simulink model "case5"  (R2024b)
settings: Solver=FixedStepAuto  StartTime=0  StopTime=1  FixedStep=1e-7  RelTol=1e-3
values from neighbouring files (symbols this model uses):
  SG_D_1_D = 0.01056    [IEEE9_case_parameters.m]    (also in case1_parameters.m; case2_parameters.m; case3_parameters.m; case4_parameters.m)
  SG_D_1_EnableSaturation = 0    [IEEE9_case_parameters.m]    (also in case1_parameters.m; case2_parameters.m; case3_parameters.m; case4_parameters.m)
  SG_D_1_f0 = 60    [IEEE9_case_parameters.m]    (also in case1_parameters.m; case2_parameters.m; case3_parameters.m; case4_parameters.m)
  SG_D_1_H = 7.5    [IEEE9_case_parameters.m]    (also in case1_parameters.m; case2_parameters.m; case3_parameters.m; case4_parameters.m)
  SG_D_1_K_A = 20    [IEEE9_case_parameters.m]    (also in case1_parameters.m; case2_parameters.m; case3_parameters.m; case4_parameters.m)
  SG_D_1_K_E = 1.000000e+1    (= 10)    [IEEE9_case_parameters.m]    (also in case1_parameters.m; case2_parameters.m; case3_parameters.m; case4_parameters.m)
  SG_D_1_K_F = 2.363    [IEEE9_case_parameters.m]    (also in case1_parameters.m; case2_parameters.m; case3_parameters.m; case4_parameters.m)
  SG_D_1_K_s = 0.5    [IEEE9_case_parameters.m]    (also in case1_parameters.m = 5; case2_parameters.m = 5; case3_parameters.m = 5; case4_parameters.m = 5)
  SG_D_1_R_a = 0.001088    [IEEE9_case_parameters.m]    (also in case1_parameters.m; case2_parameters.m; case3_parameters.m; case4_parameters.m)
  SG_D_1_S_A = 1    [IEEE9_case_parameters.m]    (also in case1_parameters.m; case2_parameters.m; case3_parameters.m; case4_parameters.m)
  SG_D_1_S_B = 0.103    [IEEE9_case_parameters.m]    (also in case1_parameters.m; case2_parameters.m; case3_parameters.m; case4_parameters.m)
  SG_D_1_S_N = 10.659857    [IEEE9_case_parameters.m]    (also in case1_parameters.m; case2_parameters.m; case3_parameters.m; case4_parameters.m)
  SG_D_1_SpeedPara = 200    [IEEE9_case_parameters.m]    (also in case1_parameters.m; case2_parameters.m; case3_parameters.m; case4_parameters.m)
  SG_D_1_T_0 = 0.720173    [IEEE9_case_parameters.m]    (also in case1_parameters.m = 0.755522; case2_parameters.m = 0.808931; case3_parameters.m = 0.869402; case4_parameters.m = 0.729316)
  SG_D_1_T_1 = 0.3    [IEEE9_case_parameters.m]    (also in case1_parameters.m; case2_parameters.m; case3_parameters.m; case4_parameters.m)
  SG_D_1_T_2 = 0.05    [IEEE9_case_parameters.m]    (also in case1_parameters.m; case2_parameters.m; case3_parameters.m; case4_parameters.m)
  SG_D_1_T_3 = 0.02    [IEEE9_case_parameters.m]    (also in case1_parameters.m; case2_parameters.m; case3_parameters.m; case4_parameters.m)
  SG_D_1_T_4 = 0.005    [IEEE9_case_parameters.m]    (also in case1_parameters.m; case2_parameters.m; case3_parameters.m; case4_parameters.m)
  SG_D_1_T_A = 0.02    [IEEE9_case_parameters.m]    (also in case1_parameters.m; case2_parameters.m; case3_parameters.m; case4_parameters.m)
  SG_D_1_T_dd = 8.000000e+0    (= 8)    [IEEE9_case_parameters.m]    (also in case1_parameters.m; case2_parameters.m; case3_parameters.m; case4_parameters.m)
  SG_D_1_T_ddd = 0.04    [IEEE9_case_parameters.m]    (also in case1_parameters.m; case2_parameters.m; case3_parameters.m; case4_parameters.m)
  SG_D_1_T_E = 0.314    [IEEE9_case_parameters.m]    (also in case1_parameters.m; case2_parameters.m; case3_parameters.m; case4_parameters.m)
  SG_D_1_T_F = 0.35    [IEEE9_case_parameters.m]    (also in case1_parameters.m; case2_parameters.m; case3_parameters.m; case4_parameters.m)
  SG_D_1_T_qd = 0.8    [IEEE9_case_parameters.m]    (also in case1_parameters.m; case2_parameters.m; case3_parameters.m; case4_parameters.m)
  SG_D_1_T_qdd = 0.02    [IEEE9_case_parameters.m]    (also in case1_parameters.m; case2_parameters.m; case3_parameters.m; case4_parameters.m)
  SG_D_1_T_speed = 0.1    [IEEE9_case_parameters.m]    (also in case1_parameters.m = 200; case2_parameters.m = 200; case3_parameters.m = 200; case4_parameters.m = 200)
  SG_D_1_T_w = 0.5    [IEEE9_case_parameters.m]    (also in case1_parameters.m; case2_parameters.m; case3_parameters.m; case4_parameters.m)
  SG_D_1_V_ref = 1.990276    [IEEE9_case_parameters.m]    (also in case1_parameters.m = 2.042296; case2_parameters.m = 2.051388; case3_parameters.m = 2.089584; case4_parameters.m = 2.01845)
  SG_D_1_w_ref = 376.991118    [IEEE9_case_parameters.m]    (also in case1_parameters.m; case2_parameters.m; case3_parameters.m; case4_parameters.m)
  SG_D_1_wb = 6.000000e+1    (= 60)    [IEEE9_case_parameters.m]    (also in case1_parameters.m; case2_parameters.m; case3_parameters.m; case4_parameters.m)
  SG_D_1_x_d = 1.9    [IEEE9_case_parameters.m]    (also in case1_parameters.m; case2_parameters.m; case3_parameters.m; case4_parameters.m)
  SG_D_1_x_dd = 0.302    [IEEE9_case_parameters.m]    (also in case1_parameters.m; case2_parameters.m; case3_parameters.m; case4_parameters.m)
  SG_D_1_x_ddd = 0.204    [IEEE9_case_parameters.m]    (also in case1_parameters.m; case2_parameters.m; case3_parameters.m; case4_parameters.m)
  SG_D_1_x_l = 0.05    [IEEE9_case_parameters.m]    (also in case1_parameters.m; case2_parameters.m; case3_parameters.m; case4_parameters.m)
  SG_D_1_x_q = 1.3    [IEEE9_case_parameters.m]    (also in case1_parameters.m; case2_parameters.m; case3_parameters.m; case4_parameters.m)
  SG_D_1_x_qd = 0.5    [IEEE9_case_parameters.m]    (also in case1_parameters.m; case2_parameters.m; case3_parameters.m; case4_parameters.m)
  SG_D_1_x_qdd = 0.3    [IEEE9_case_parameters.m]    (also in case1_parameters.m; case2_parameters.m; case3_parameters.m; case4_parameters.m)
  SG_D_2_D = 0.02    [IEEE9_case_parameters.m]    (also in case1_parameters.m; case2_parameters.m; case3_parameters.m; case4_parameters.m)
  SG_D_2_EnableSaturation = 0    [IEEE9_case_parameters.m]    (also in case1_parameters.m; case2_parameters.m; case3_parameters.m; case4_parameters.m)
  SG_D_2_f0 = 60    [IEEE9_case_parameters.m]    (also in case1_parameters.m; case2_parameters.m; case3_parameters.m; case4_parameters.m)
  SG_D_2_H = 8.000000e+0    (= 8)    [IEEE9_case_parameters.m]    (also in case1_parameters.m; case2_parameters.m; case3_parameters.m; case4_parameters.m)
  SG_D_2_K_A = 20    [IEEE9_case_parameters.m]    (also in case1_parameters.m; case2_parameters.m; case3_parameters.m; case4_parameters.m)
  SG_D_2_K_E = 1.000000e+1    (= 10)    [IEEE9_case_parameters.m]    (also in case1_parameters.m; case2_parameters.m; case3_parameters.m; case4_parameters.m)
  SG_D_2_K_F = 2.363    [IEEE9_case_parameters.m]    (also in case1_parameters.m; case2_parameters.m; case3_parameters.m; case4_parameters.m)
  SG_D_2_K_s = 0.5    [IEEE9_case_parameters.m]    (also in case1_parameters.m = 4; case2_parameters.m = 4; case3_parameters.m = 4; case4_parameters.m = 4)
  SG_D_2_R_a = 0.001088    [IEEE9_case_parameters.m]    (also in case1_parameters.m; case2_parameters.m; case3_parameters.m; case4_parameters.m)
  SG_D_2_S_A = 1    [IEEE9_case_parameters.m]    (also in case1_parameters.m; case2_parameters.m; case3_parameters.m; case4_parameters.m)
  SG_D_2_S_B = 0.103    [IEEE9_case_parameters.m]    (also in case1_parameters.m; case2_parameters.m; case3_parameters.m; case4_parameters.m)
  SG_D_2_S_N = 10.659857    [IEEE9_case_parameters.m]    (also in case1_parameters.m; case2_parameters.m; case3_parameters.m; case4_parameters.m)
  SG_D_2_SpeedPara = 200    [IEEE9_case_parameters.m]    (also in case1_parameters.m; case2_parameters.m; case3_parameters.m; case4_parameters.m)
  SG_D_2_T_0 = 1.632913    [IEEE9_case_parameters.m]    (also in case1_parameters.m = 1.632925; case2_parameters.m = 1.632915; case3_parameters.m = 1.632914; case4_parameters.m = 1.632927)
  SG_D_2_T_1 = 0.2    [IEEE9_case_parameters.m]    (also in case1_parameters.m; case2_parameters.m; case3_parameters.m; case4_parameters.m)
  SG_D_2_T_2 = 0.05    [IEEE9_case_parameters.m]    (also in case1_parameters.m; case2_parameters.m; case3_parameters.m; case4_parameters.m)
  SG_D_2_T_3 = 0.02    [IEEE9_case_parameters.m]    (also in case1_parameters.m; case2_parameters.m; case3_parameters.m; case4_parameters.m)
  SG_D_2_T_4 = 0.005    [IEEE9_case_parameters.m]    (also in case1_parameters.m; case2_parameters.m; case3_parameters.m; case4_parameters.m)
  SG_D_2_T_A = 0.02    [IEEE9_case_parameters.m]    (also in case1_parameters.m; case2_parameters.m; case3_parameters.m; case4_parameters.m)
  SG_D_2_T_dd = 7.9    [IEEE9_case_parameters.m]    (also in case1_parameters.m; case2_parameters.m; case3_parameters.m; case4_parameters.m)
  SG_D_2_T_ddd = 0.04    [IEEE9_case_parameters.m]    (also in case1_parameters.m; case2_parameters.m; case3_parameters.m; case4_parameters.m)
  SG_D_2_T_E = 0.314    [IEEE9_case_parameters.m]    (also in case1_parameters.m; case2_parameters.m; case3_parameters.m; case4_parameters.m)
  SG_D_2_T_F = 0.35    [IEEE9_case_parameters.m]    (also in case1_parameters.m; case2_parameters.m; case3_parameters.m; case4_parameters.m)
  SG_D_2_T_qd = 0.8    [IEEE9_case_parameters.m]    (also in case1_parameters.m; case2_parameters.m; case3_parameters.m; case4_parameters.m)
  SG_D_2_T_qdd = 0.015    [IEEE9_case_parameters.m]    (also in case1_parameters.m; case2_parameters.m; case3_parameters.m; case4_parameters.m)
  SG_D_2_T_speed = 0.1    [IEEE9_case_parameters.m]    (also in case1_parameters.m = 150; case2_parameters.m = 150; case3_parameters.m = 150; case4_parameters.m = 150)
  SG_D_2_T_w = 0.35    [IEEE9_case_parameters.m]    (also in case1_parameters.m; case2_parameters.m; case3_parameters.m; case4_parameters.m)
  SG_D_2_V_ref = 2.58547    [IEEE9_case_parameters.m]    (also in case1_parameters.m = 2.597896; case2_parameters.m = 2.587136; case3_parameters.m = 2.586042; case4_parameters.m = 2.599679)
  SG_D_2_w_ref = 376.991118    [IEEE9_case_parameters.m]    (also in case1_parameters.m; case2_parameters.m; case3_parameters.m; case4_parameters.m)
  SG_D_2_wb = 6.000000e+1    (= 60)    [IEEE9_case_parameters.m]    (also in case1_parameters.m; case2_parameters.m; case3_parameters.m; case4_parameters.m)
  SG_D_2_x_d = 1.8    [IEEE9_case_parameters.m]    (also in case1_parameters.m; case2_parameters.m; case3_parameters.m; case4_parameters.m)
  SG_D_2_x_dd = 0.302    [IEEE9_case_parameters.m]    (also in case1_parameters.m; case2_parameters.m; case3_parameters.m; case4_parameters.m)
  SG_D_2_x_ddd = 0.204    [IEEE9_case_parameters.m]    (also in case1_parameters.m; case2_parameters.m; case3_parameters.m; case4_parameters.m)
  SG_D_2_x_l = 0.05    [IEEE9_case_parameters.m]    (also in case1_parameters.m; case2_parameters.m; case3_parameters.m; case4_parameters.m)
  SG_D_2_x_q = 1.25    [IEEE9_case_parameters.m]    (also in case1_parameters.m; case2_parameters.m; case3_parameters.m; case4_parameters.m)
  SG_D_2_x_qd = 0.5    [IEEE9_case_parameters.m]    (also in case1_parameters.m; case2_parameters.m; case3_parameters.m; case4_parameters.m)
  SG_D_2_x_qdd = 0.3    [IEEE9_case_parameters.m]    (also in case1_parameters.m; case2_parameters.m; case3_parameters.m; case4_parameters.m)
  SG_D_3_D = 0.02    [IEEE9_case_parameters.m]    (also in case1_parameters.m; case2_parameters.m; case3_parameters.m; case4_parameters.m)
  SG_D_3_EnableSaturation = 0    [IEEE9_case_parameters.m]    (also in case1_parameters.m; case2_parameters.m; case3_parameters.m; case4_parameters.m)
  SG_D_3_f0 = 60    [IEEE9_case_parameters.m]    (also in case1_parameters.m; case2_parameters.m; case3_parameters.m; case4_parameters.m)
  SG_D_3_H = 7.7    [IEEE9_case_parameters.m]    (also in case1_parameters.m; case2_parameters.m; case3_parameters.m; case4_parameters.m)
  SG_D_3_K_A = 20    [IEEE9_case_parameters.m]    (also in case1_parameters.m; case2_parameters.m; case3_parameters.m; case4_parameters.m)
  SG_D_3_K_E = 1.000000e+1    (= 10)    [IEEE9_case_parameters.m]    (also in case1_parameters.m; case2_parameters.m; case3_parameters.m; case4_parameters.m)
  SG_D_3_K_F = 2.363    [IEEE9_case_parameters.m]    (also in case1_parameters.m; case2_parameters.m; case3_parameters.m; case4_parameters.m)
  SG_D_3_K_s = 0.2    [IEEE9_case_parameters.m]    (also in case1_parameters.m = 2; case2_parameters.m = 2; case3_parameters.m = 2; case4_parameters.m = 2)
  SG_D_3_R_a = 0.001088    [IEEE9_case_parameters.m]    (also in case1_parameters.m; case2_parameters.m; case3_parameters.m; case4_parameters.m)
  SG_D_3_S_A = 1    [IEEE9_case_parameters.m]    (also in case1_parameters.m; case2_parameters.m; case3_parameters.m; case4_parameters.m)
  SG_D_3_S_B = 0.103    [IEEE9_case_parameters.m]    (also in case1_parameters.m; case2_parameters.m; case3_parameters.m; case4_parameters.m)
  SG_D_3_S_N = 10.659857    [IEEE9_case_parameters.m]    (also in case1_parameters.m; case2_parameters.m; case3_parameters.m; case4_parameters.m)
  SG_D_3_SpeedPara = 200    [IEEE9_case_parameters.m]    (also in case1_parameters.m; case2_parameters.m; case3_parameters.m; case4_parameters.m)
  SG_D_3_T_0 = 0.850788    [IEEE9_case_parameters.m]    (also in case1_parameters.m = 0.850786; case2_parameters.m = 0.850787; case3_parameters.m; case4_parameters.m = 0.850786)
  SG_D_3_T_1 = 0.2    [IEEE9_case_parameters.m]    (also in case1_parameters.m; case2_parameters.m; case3_parameters.m; case4_parameters.m)
  SG_D_3_T_2 = 0.05    [IEEE9_case_parameters.m]    (also in case1_parameters.m; case2_parameters.m; case3_parameters.m; case4_parameters.m)
  SG_D_3_T_3 = 0.02    [IEEE9_case_parameters.m]    (also in case1_parameters.m; case2_parameters.m; case3_parameters.m; case4_parameters.m)
  SG_D_3_T_4 = 0.005    [IEEE9_case_parameters.m]    (also in case1_parameters.m; case2_parameters.m; case3_parameters.m; case4_parameters.m)
  SG_D_3_T_A = 0.02    [IEEE9_case_parameters.m]    (also in case1_parameters.m; case2_parameters.m; case3_parameters.m; case4_parameters.m)
  SG_D_3_T_dd = 8.1    [IEEE9_case_parameters.m]    (also in case1_parameters.m; case2_parameters.m; case3_parameters.m; case4_parameters.m)
  SG_D_3_T_ddd = 0.04    [IEEE9_case_parameters.m]    (also in case1_parameters.m; case2_parameters.m; case3_parameters.m; case4_parameters.m)
  SG_D_3_T_E = 0.314    [IEEE9_case_parameters.m]    (also in case1_parameters.m; case2_parameters.m; case3_parameters.m; case4_parameters.m)
  SG_D_3_T_F = 0.35    [IEEE9_case_parameters.m]    (also in case1_parameters.m; case2_parameters.m; case3_parameters.m; case4_parameters.m)
  SG_D_3_T_qd = 0.8    [IEEE9_case_parameters.m]    (also in case1_parameters.m; case2_parameters.m; case3_parameters.m; case4_parameters.m)
  SG_D_3_T_qdd = 0.015    [IEEE9_case_parameters.m]    (also in case1_parameters.m; case2_parameters.m; case3_parameters.m; case4_parameters.m)
  SG_D_3_T_speed = 0.1    [IEEE9_case_parameters.m]    (also in case1_parameters.m = 180; case2_parameters.m = 180; case3_parameters.m = 180; case4_parameters.m = 180)
  SG_D_3_T_w = 0.4    [IEEE9_case_parameters.m]    (also in case1_parameters.m; case2_parameters.m; case3_parameters.m; case4_parameters.m)
  SG_D_3_V_ref = 1.892727    [IEEE9_case_parameters.m]    (also in case1_parameters.m = 1.906439; case2_parameters.m = 1.895535; case3_parameters.m = 1.892105; case4_parameters.m = 1.906598)
  SG_D_3_w_ref = 376.991118    [IEEE9_case_parameters.m]    (also in case1_parameters.m; case2_parameters.m; case3_parameters.m; case4_parameters.m)
  SG_D_3_wb = 6.000000e+1    (= 60)    [IEEE9_case_parameters.m]    (also in case1_parameters.m; case2_parameters.m; case3_parameters.m; case4_parameters.m)
  SG_D_3_x_d = 1.85    [IEEE9_case_parameters.m]    (also in case1_parameters.m; case2_parameters.m; case3_parameters.m; case4_parameters.m)
  SG_D_3_x_dd = 0.302    [IEEE9_case_parameters.m]    (also in case1_parameters.m; case2_parameters.m; case3_parameters.m; case4_parameters.m)
  SG_D_3_x_ddd = 0.204    [IEEE9_case_parameters.m]    (also in case1_parameters.m; case2_parameters.m; case3_parameters.m; case4_parameters.m)
  SG_D_3_x_l = 0.05    [IEEE9_case_parameters.m]    (also in case1_parameters.m; case2_parameters.m; case3_parameters.m; case4_parameters.m)
  SG_D_3_x_q = 1.2    [IEEE9_case_parameters.m]    (also in case1_parameters.m; case2_parameters.m; case3_parameters.m; case4_parameters.m)
  SG_D_3_x_qd = 0.5    [IEEE9_case_parameters.m]    (also in case1_parameters.m; case2_parameters.m; case3_parameters.m; case4_parameters.m)
  SG_D_3_x_qdd = 0.3    [IEEE9_case_parameters.m]    (also in case1_parameters.m; case2_parameters.m; case3_parameters.m; case4_parameters.m)
(part 2 of 12)

== system case5/SG_D_2 ==
  v_d_SG_D_2 : Inport
  v_q_SG_D_2 : Inport  Port=2
  E_fd_SG_D_2 : Integrator  InitialCondition=3.1862497744439606
  Px_1_SG_D_2 : Integrator  InitialCondition=0.0
  Px_2_SG_D_2 : Integrator  InitialCondition=0.0
  Px_3_SG_D_2 : Integrator  InitialCondition=6.670039757612852e-24
  R_f_SG_D_2 : Integrator  InitialCondition=21.5117377628888
  T_e_SG_D_2_block : Subsystem
  T_m_SG_D_2 : Integrator  InitialCondition=1.6329204678673217
  V_f_SG_D_2 : Integrator  InitialCondition=31.862497744439608
  d_E_fd_SG_D_2_block : Subsystem
  d_Px_1_SG_D_2_block : Subsystem
  d_Px_2_SG_D_2_block : Subsystem
  d_Px_3_SG_D_2_block : Subsystem
  d_R_f_SG_D_2_block : Subsystem
  d_T_m_SG_D_2_block : Subsystem
  d_V_f_SG_D_2_block : Subsystem
  d_psi_1d_SG_D_2_block : Subsystem
  d_psi_d_SG_D_2_block : Subsystem
  d_psi_fd_SG_D_2_block : Subsystem
  d_psi_gq_SG_D_2_block : Subsystem
  d_psi_kq_SG_D_2_block : Subsystem
  d_psi_q_SG_D_2_block : Subsystem
  d_theta_SG_D_2_block : Subsystem
  d_w_SG_D_2_block : Subsystem
  i_d_SG_D_2_block : Subsystem
  i_q_SG_D_2_block : Subsystem
  psi_1d_SG_D_2 : Integrator  InitialCondition=0.5852448096125112
  psi_d_SG_D_2 : Integrator  InitialCondition=0.5109303820458982
  psi_fd_SG_D_2 : Integrator  InitialCondition=0.95978952454824
  psi_gq_SG_D_2 : Integrator  InitialCondition=0.5170107087646497
  psi_kq_SG_D_2 : Integrator  InitialCondition=-0.8272171340234395
  psi_q_SG_D_2 : Integrator  InitialCondition=-0.8616845146077495
  theta_SG_D_2 : Integrator  InitialCondition=1.2193477459639033
  theta_SG_D_2_out_block : Subsystem
  w_SG_D_2 : Integrator  InitialCondition=376.99111843077515
  w_SG_D_2_out_block : Subsystem
  i_d_SG_D_2 : Outport
  i_q_SG_D_2 : Outport  Port=2
  T_e_SG_D_2 : Outport  Port=3
  w_SG_D_2_out : Outport  Port=4
  theta_SG_D_2_out : Outport  Port=5
  wires:
  d_T_m_SG_D_2_block/1(Blockout_d_T_m_SG_D_2_8be19) -> T_m_SG_D_2/1
  T_e_SG_D_2_block/1(Blockout_T_e_SG_D_2_32ea4) -> T_e_SG_D_2/1
  d_Px_2_SG_D_2_block/1(Blockout_d_Px_2_SG_D_2_04e36) -> Px_2_SG_D_2/1
  w_SG_D_2/1 -> d_psi_q_SG_D_2_block/9(State_w_SG_D_2_ff297), d_psi_d_SG_D_2_block/9(State_w_SG_D_2_93911), d_w_SG_D_2_block/1(State_w_SG_D_2_6739b), d_V_f_SG_D_2_block/8(State_w_SG_D_2_0ea60), d_V_f_SG_D_2_block/13(State_w_SG_D_2_f8832), d_theta_SG_D_2_block/1(State_w_SG_D_2_4ff61), d_T_m_SG_D_2_block/1(State_w_SG_D_2_ee856), d_Px_2_SG_D_2_block/4(State_w_SG_D_2_c4bce), d_Px_3_SG_D_2_block/6(State_w_SG_D_2_e9070), d_Px_1_SG_D_2_block/2(State_w_SG_D_2_0a872), w_SG_D_2_out_block/1(State_w_SG_D_2_5e653)
  d_Px_1_SG_D_2_block/1(Blockout_d_Px_1_SG_D_2_3a836) -> Px_1_SG_D_2/1
  d_theta_SG_D_2_block/1(Blockout_d_theta_SG_D_2_f9fe2) -> theta_SG_D_2/1
  psi_q_SG_D_2/1 -> d_psi_d_SG_D_2_block/8(State_psi_q_SG_D_2_39081), d_psi_gq_SG_D_2_block/9(State_psi_q_SG_D_2_8da15), d_psi_kq_SG_D_2_block/5(State_psi_q_SG_D_2_342e1), d_psi_gq_SG_D_2_block/6(State_psi_q_SG_D_2_ffa91), d_w_SG_D_2_block/6(State_psi_q_SG_D_2_d0bfc), d_V_f_SG_D_2_block/7(State_psi_q_SG_D_2_3f571), d_V_f_SG_D_2_block/11(State_psi_q_SG_D_2_64f5f), i_q_SG_D_2_block/3(State_psi_q_SG_D_2_28683), d_w_SG_D_2_block/7(State_psi_q_SG_D_2_59cd6), d_psi_q_SG_D_2_block/3(State_psi_q_SG_D_2_48ee2), T_e_SG_D_2_block/4(State_psi_q_SG_D_2_7d7d0), T_e_SG_D_2_block/5(State_psi_q_SG_D_2_860cc), i_d_SG_D_2_block/3(State_psi_q_SG_D_2_2fd58)
  w_SG_D_2_out_block/1(Blockout_w_SG_D_2_out_edd03) -> w_SG_D_2_out/1
  d_Px_3_SG_D_2_block/1(Blockout_d_Px_3_SG_D_2_0e921) -> Px_3_SG_D_2/1
  psi_gq_SG_D_2/1 -> d_psi_q_SG_D_2_block/1(State_psi_gq_SG_D_2_56d9a), d_psi_gq_SG_D_2_block/1(State_psi_gq_SG_D_2_87c46), d_psi_gq_SG_D_2_block/2(State_psi_gq_SG_D_2_c98fa), d_psi_gq_SG_D_2_block/4(State_psi_gq_SG_D_2_58af0), d_psi_kq_SG_D_2_block/3(State_psi_gq_SG_D_2_50e2d), d_w_SG_D_2_block/4(State_psi_gq_SG_D_2_c0fca), d_psi_gq_SG_D_2_block/7(State_psi_gq_SG_D_2_c3a0a), i_d_SG_D_2_block/1(State_psi_gq_SG_D_2_2f279), d_psi_kq_SG_D_2_block/1(State_psi_gq_SG_D_2_a995b), i_q_SG_D_2_block/1(State_psi_gq_SG_D_2_27a63), d_V_f_SG_D_2_block/9(State_psi_gq_SG_D_2_79d5b), T_e_SG_D_2_block/2(State_psi_gq_SG_D_2_1f7cf)
  psi_fd_SG_D_2/1 -> d_psi_fd_SG_D_2_block/2(State_psi_fd_SG_D_2_52249), d_psi_fd_SG_D_2_block/4(State_psi_fd_SG_D_2_bd521), d_psi_fd_SG_D_2_block/10(State_psi_fd_SG_D_2_29cbb), d_psi_fd_SG_D_2_block/7(State_psi_fd_SG_D_2_2448d), d_psi_d_SG_D_2_block/3(State_psi_fd_SG_D_2_ff9ed), d_V_f_SG_D_2_block/6(State_psi_fd_SG_D_2_d94f6), d_psi_1d_SG_D_2_block/2(State_psi_fd_SG_D_2_ecfb2), i_d_SG_D_2_block/7(State_psi_fd_SG_D_2_ae8c9), d_w_SG_D_2_block/10(State_psi_fd_SG_D_2_d0345), d_psi_1d_SG_D_2_block/5(State_psi_fd_SG_D_2_f55be), i_q_SG_D_2_block/7(State_psi_fd_SG_D_2_80ec4), T_e_SG_D_2_block/8(State_psi_fd_SG_D_2_f288a)
  psi_kq_SG_D_2/1 -> d_V_f_SG_D_2_block/10(State_psi_kq_SG_D_2_dc614), d_w_SG_D_2_block/5(State_psi_kq_SG_D_2_46ea8), d_psi_gq_SG_D_2_block/5(State_psi_kq_SG_D_2_220dd), d_psi_kq_SG_D_2_block/4(State_psi_kq_SG_D_2_80926), i_d_SG_D_2_block/2(State_psi_kq_SG_D_2_3a555), d_psi_gq_SG_D_2_block/8(State_psi_kq_SG_D_2_f5814), d_psi_q_SG_D_2_block/2(State_psi_kq_SG_D_2_66775), i_q_SG_D_2_block/2(State_psi_kq_SG_D_2_d20f4), d_psi_gq_SG_D_2_block/3(State_psi_kq_SG_D_2_803f1), T_e_SG_D_2_block/3(State_psi_kq_SG_D_2_b1f64), d_psi_kq_SG_D_2_block/2(State_psi_kq_SG_D_2_e8f3b)
  psi_1d_SG_D_2/1 -> d_psi_fd_SG_D_2_block/3(State_psi_1d_SG_D_2_569a8), d_psi_fd_SG_D_2_block/5(State_psi_1d_SG_D_2_de869), d_psi_fd_SG_D_2_block/8(State_psi_1d_SG_D_2_50b72), d_psi_d_SG_D_2_block/1(State_psi_1d_SG_D_2_04eff), d_psi_1d_SG_D_2_block/3(State_psi_1d_SG_D_2_31dd9), d_w_SG_D_2_block/8(State_psi_1d_SG_D_2_f1571), d_V_f_SG_D_2_block/4(State_psi_1d_SG_D_2_e8660), i_d_SG_D_2_block/5(State_psi_1d_SG_D_2_aa18d), i_q_SG_D_2_block/5(State_psi_1d_SG_D_2_19eb0), T_e_SG_D_2_block/6(State_psi_1d_SG_D_2_4989b), d_psi_1d_SG_D_2_block/1(State_psi_1d_SG_D_2_febab)
  Px_1_SG_D_2/1 -> d_Px_3_SG_D_2_block/4(State_Px_1_SG_D_2_820be), d_Px_1_SG_D_2_block/1(State_Px_1_SG_D_2_dcfec), d_Px_3_SG_D_2_block/5(State_Px_1_SG_D_2_81adf), d_Px_2_SG_D_2_block/3(State_Px_1_SG_D_2_6b838), d_Px_2_SG_D_2_block/2(State_Px_1_SG_D_2_e7928)
  theta_SG_D_2/1 -> d_psi_d_SG_D_2_block/5(State_theta_SG_D_2_47dce), d_psi_d_SG_D_2_block/7(State_theta_SG_D_2_18c28), i_d_SG_D_2_block/4(State_theta_SG_D_2_e2546), i_q_SG_D_2_block/4(State_theta_SG_D_2_24bbd), d_psi_q_SG_D_2_block/5(State_theta_SG_D_2_953f6), i_q_SG_D_2_block/8(State_theta_SG_D_2_e7cf1), i_d_SG_D_2_block/8(State_theta_SG_D_2_a5f3d), d_psi_q_SG_D_2_block/7(State_theta_SG_D_2_428e6), theta_SG_D_2_out_block/1(State_theta_SG_D_2_369d6)
  Px_2_SG_D_2/1 -> d_Px_3_SG_D_2_block/2(State_Px_2_SG_D_2_ea741), d_Px_2_SG_D_2_block/1(State_Px_2_SG_D_2_3d84e), d_Px_3_SG_D_2_block/3(State_Px_2_SG_D_2_55edc)
  v_d_SG_D_2/1 -> d_psi_d_SG_D_2_block/4(Input_v_d_SG_D_2_e8182), d_psi_q_SG_D_2_block/4(Input_v_d_SG_D_2_6ca72)
  i_d_SG_D_2_block/1(Blockout_i_d_SG_D_2_72f47) -> i_d_SG_D_2/1
  psi_d_SG_D_2/1 -> d_psi_fd_SG_D_2_block/6(State_psi_d_SG_D_2_2ae43), d_psi_d_SG_D_2_block/2(State_psi_d_SG_D_2_38234), d_psi_1d_SG_D_2_block/4(State_psi_d_SG_D_2_bbb49), d_V_f_SG_D_2_block/12(State_psi_d_SG_D_2_2ef51), d_V_f_SG_D_2_block/5(State_psi_d_SG_D_2_250ba), d_psi_q_SG_D_2_block/8(State_psi_d_SG_D_2_a68ec), d_w_SG_D_2_block/9(State_psi_d_SG_D_2_c4658), i_d_SG_D_2_block/6(State_psi_d_SG_D_2_3866e), T_e_SG_D_2_block/1(State_psi_d_SG_D_2_8764f), d_w_SG_D_2_block/3(State_psi_d_SG_D_2_c40be), d_psi_fd_SG_D_2_block/9(State_psi_d_SG_D_2_60bb1), i_q_SG_D_2_block/6(State_psi_d_SG_D_2_881d1), T_e_SG_D_2_block/7(State_psi_d_SG_D_2_cc96c)
  d_V_f_SG_D_2_block/1(Blockout_d_V_f_SG_D_2_8ab92) -> V_f_SG_D_2/1
  v_q_SG_D_2/1 -> d_psi_d_SG_D_2_block/6(Input_v_q_SG_D_2_617bb), d_psi_q_SG_D_2_block/6(Input_v_q_SG_D_2_c1f9e)
  T_m_SG_D_2/1 -> d_T_m_SG_D_2_block/2(State_T_m_SG_D_2_0b68a), d_w_SG_D_2_block/2(State_T_m_SG_D_2_a5b2e)
  R_f_SG_D_2/1 -> d_R_f_SG_D_2_block/2(State_R_f_SG_D_2_625bf), d_V_f_SG_D_2_block/2(State_R_f_SG_D_2_30619)
  theta_SG_D_2_out_block/1(Blockout_theta_SG_D_2_out_abd77) -> theta_SG_D_2_out/1
  d_psi_kq_SG_D_2_block/1(Blockout_d_psi_kq_SG_D_2_70fc6) -> psi_kq_SG_D_2/1
  d_R_f_SG_D_2_block/1(Blockout_d_R_f_SG_D_2_818dd) -> R_f_SG_D_2/1
  d_psi_gq_SG_D_2_block/1(Blockout_d_psi_gq_SG_D_2_29e5c) -> psi_gq_SG_D_2/1
  d_psi_1d_SG_D_2_block/1(Blockout_d_psi_1d_SG_D_2_44b96) -> psi_1d_SG_D_2/1
  d_psi_q_SG_D_2_block/1(Blockout_d_psi_q_SG_D_2_3921f) -> psi_q_SG_D_2/1
  d_psi_d_SG_D_2_block/1(Blockout_d_psi_d_SG_D_2_c5ec0) -> psi_d_SG_D_2/1
  d_w_SG_D_2_block/1(Blockout_d_w_SG_D_2_3d116) -> w_SG_D_2/1
  i_q_SG_D_2_block/1(Blockout_i_q_SG_D_2_ddca7) -> i_q_SG_D_2/1
  V_f_SG_D_2/1 -> d_V_f_SG_D_2_block/14(State_V_f_SG_D_2_95214), d_E_fd_SG_D_2_block/2(State_V_f_SG_D_2_4e077)
  Px_3_SG_D_2/1 -> d_V_f_SG_D_2_block/3(State_Px_3_SG_D_2_b4828), d_Px_3_SG_D_2_block/1(State_Px_3_SG_D_2_615b8)
  d_E_fd_SG_D_2_block/1(Blockout_d_E_fd_SG_D_2_55c73) -> E_fd_SG_D_2/1
  E_fd_SG_D_2/1 -> d_V_f_SG_D_2_block/1(State_E_fd_SG_D_2_ced48), d_R_f_SG_D_2_block/1(State_E_fd_SG_D_2_65d60), d_E_fd_SG_D_2_block/1(State_E_fd_SG_D_2_808fd), d_psi_fd_SG_D_2_block/1(State_E_fd_SG_D_2_4bfea)
  d_psi_fd_SG_D_2_block/1(Blockout_d_psi_fd_SG_D_2_6ca49) -> psi_fd_SG_D_2/1

== system case5/SG_D_3 ==
  v_d_SG_D_3 : Inport
  v_q_SG_D_3 : Inport  Port=2
  E_fd_SG_D_3 : Integrator  InitialCondition=1.7984887709053456
  Px_1_SG_D_3 : Integrator  InitialCondition=0.0
  Px_2_SG_D_3 : Integrator  InitialCondition=0.0
  Px_3_SG_D_3 : Integrator  InitialCondition=-1.4673797984671398e-24
  R_f_SG_D_3 : Integrator  InitialCondition=12.142368473283806
  T_e_SG_D_3_block : Subsystem
  T_m_SG_D_3 : Integrator  InitialCondition=0.8507866955563819
  V_f_SG_D_3 : Integrator  InitialCondition=17.984887709053456
  d_E_fd_SG_D_3_block : Subsystem
  d_Px_1_SG_D_3_block : Subsystem
  d_Px_2_SG_D_3_block : Subsystem
  d_Px_3_SG_D_3_block : Subsystem
  d_R_f_SG_D_3_block : Subsystem
  d_T_m_SG_D_3_block : Subsystem
  d_V_f_SG_D_3_block : Subsystem
  d_psi_1d_SG_D_3_block : Subsystem
  d_psi_d_SG_D_3_block : Subsystem
  d_psi_fd_SG_D_3_block : Subsystem
  d_psi_gq_SG_D_3_block : Subsystem
  d_psi_kq_SG_D_3_block : Subsystem
  d_psi_q_SG_D_3_block : Subsystem
  d_theta_SG_D_3_block : Subsystem
  d_w_SG_D_3_block : Subsystem
  i_d_SG_D_3_block : Subsystem
  i_q_SG_D_3_block : Subsystem
  psi_1d_SG_D_3 : Integrator  InitialCondition=0.7206007980275798
  psi_d_SG_D_3 : Integrator  InitialCondition=0.6906594654476417
  psi_fd_SG_D_3 : Integrator  InitialCondition=0.8715051142304671
  psi_gq_SG_D_3 : Integrator  InitialCondition=0.4226007274570196
  psi_kq_SG_D_3 : Integrator  InitialCondition=-0.6942726236793892
  psi_q_SG_D_3 : Integrator  InitialCondition=-0.7244583899263193
  theta_SG_D_3 : Integrator  InitialCondition=0.9043269566391599
  theta_SG_D_3_out_block : Subsystem
  w_SG_D_3 : Integrator  InitialCondition=376.99111843077515
  w_SG_D_3_out_block : Subsystem
  i_d_SG_D_3 : Outport
  i_q_SG_D_3 : Outport  Port=2
  T_e_SG_D_3 : Outport  Port=3
  w_SG_D_3_out : Outport  Port=4
  theta_SG_D_3_out : Outport  Port=5
  wires:
  d_Px_1_SG_D_3_block/1(Blockout_d_Px_1_SG_D_3_9be4e) -> Px_1_SG_D_3/1
  w_SG_D_3/1 -> d_psi_d_SG_D_3_block/9(State_w_SG_D_3_5916e), d_w_SG_D_3_block/1(State_w_SG_D_3_c3b06), d_V_f_SG_D_3_block/8(State_w_SG_D_3_90604), d_psi_q_SG_D_3_block/9(State_w_SG_D_3_7587a), d_V_f_SG_D_3_block/13(State_w_SG_D_3_d21e8), d_theta_SG_D_3_block/1(State_w_SG_D_3_3c4ab), d_T_m_SG_D_3_block/1(State_w_SG_D_3_0ca8a), d_Px_1_SG_D_3_block/2(State_w_SG_D_3_220ce), d_Px_2_SG_D_3_block/4(State_w_SG_D_3_ac5cc), d_Px_3_SG_D_3_block/6(State_w_SG_D_3_03b1d), w_SG_D_3_out_block/1(State_w_SG_D_3_fee15)
  d_T_m_SG_D_3_block/1(Blockout_d_T_m_SG_D_3_d3830) -> T_m_SG_D_3/1
  d_w_SG_D_3_block/1(Blockout_d_w_SG_D_3_cf3fb) -> w_SG_D_3/1
  Px_1_SG_D_3/1 -> d_Px_3_SG_D_3_block/4(State_Px_1_SG_D_3_769ed), d_Px_2_SG_D_3_block/3(State_Px_1_SG_D_3_6c166), d_Px_2_SG_D_3_block/2(State_Px_1_SG_D_3_ebea2), d_Px_3_SG_D_3_block/5(State_Px_1_SG_D_3_ab3a0), d_Px_1_SG_D_3_block/1(State_Px_1_SG_D_3_e9303)
  d_theta_SG_D_3_block/1(Blockout_d_theta_SG_D_3_6d326) -> theta_SG_D_3/1
  Px_2_SG_D_3/1 -> d_Px_2_SG_D_3_block/1(State_Px_2_SG_D_3_b50b4), d_Px_3_SG_D_3_block/2(State_Px_2_SG_D_3_8f252), d_Px_3_SG_D_3_block/3(State_Px_2_SG_D_3_5d3da)
  d_Px_3_SG_D_3_block/1(Blockout_d_Px_3_SG_D_3_07f5b) -> Px_3_SG_D_3/1
  R_f_SG_D_3/1 -> d_V_f_SG_D_3_block/2(State_R_f_SG_D_3_65c10), d_R_f_SG_D_3_block/2(State_R_f_SG_D_3_2ac4f)
  w_SG_D_3_out_block/1(Blockout_w_SG_D_3_out_017ab) -> w_SG_D_3_out/1
  d_Px_2_SG_D_3_block/1(Blockout_d_Px_2_SG_D_3_d6435) -> Px_2_SG_D_3/1
  T_m_SG_D_3/1 -> d_T_m_SG_D_3_block/2(State_T_m_SG_D_3_db6e5), d_w_SG_D_3_block/2(State_T_m_SG_D_3_e3476)
  v_d_SG_D_3/1 -> d_psi_q_SG_D_3_block/4(Input_v_d_SG_D_3_84d49), d_psi_d_SG_D_3_block/4(Input_v_d_SG_D_3_606f6)
  v_q_SG_D_3/1 -> d_psi_d_SG_D_3_block/6(Input_v_q_SG_D_3_a4294), d_psi_q_SG_D_3_block/6(Input_v_q_SG_D_3_69553)
  psi_kq_SG_D_3/1 -> d_psi_q_SG_D_3_block/2(State_psi_kq_SG_D_3_924ec), d_psi_gq_SG_D_3_block/3(State_psi_kq_SG_D_3_58aa9), d_psi_gq_SG_D_3_block/5(State_psi_kq_SG_D_3_80c97), d_psi_kq_SG_D_3_block/4(State_psi_kq_SG_D_3_7e333), d_w_SG_D_3_block/5(State_psi_kq_SG_D_3_92701), d_V_f_SG_D_3_block/10(State_psi_kq_SG_D_3_31833), i_d_SG_D_3_block/2(State_psi_kq_SG_D_3_2d375), d_psi_kq_SG_D_3_block/2(State_psi_kq_SG_D_3_1fc99), T_e_SG_D_3_block/3(State_psi_kq_SG_D_3_f2804), i_q_SG_D_3_block/2(State_psi_kq_SG_D_3_73f11), d_psi_gq_SG_D_3_block/8(State_psi_kq_SG_D_3_d3364)
  theta_SG_D_3/1 -> d_psi_d_SG_D_3_block/5(State_theta_SG_D_3_c5e42), d_psi_q_SG_D_3_block/7(State_theta_SG_D_3_ee4f0), i_d_SG_D_3_block/8(State_theta_SG_D_3_5a6b6), i_q_SG_D_3_block/4(State_theta_SG_D_3_ec54c), i_d_SG_D_3_block/4(State_theta_SG_D_3_03d7d), d_psi_q_SG_D_3_block/5(State_theta_SG_D_3_74150), i_q_SG_D_3_block/8(State_theta_SG_D_3_27a42), d_psi_d_SG_D_3_block/7(State_theta_SG_D_3_aedc7), theta_SG_D_3_out_block/1(State_theta_SG_D_3_f776d)
  psi_d_SG_D_3/1 -> d_psi_fd_SG_D_3_block/6(State_psi_d_SG_D_3_99e22), d_psi_fd_SG_D_3_block/9(State_psi_d_SG_D_3_9a2c9), d_psi_d_SG_D_3_block/2(State_psi_d_SG_D_3_d393d), d_psi_q_SG_D_3_block/8(State_psi_d_SG_D_3_b8185), d_psi_1d_SG_D_3_block/4(State_psi_d_SG_D_3_3e3a9), d_w_SG_D_3_block/9(State_psi_d_SG_D_3_9af62), d_V_f_SG_D_3_block/12(State_psi_d_SG_D_3_26750), i_d_SG_D_3_block/6(State_psi_d_SG_D_3_22276), d_V_f_SG_D_3_block/5(State_psi_d_SG_D_3_3db68), i_q_SG_D_3_block/6(State_psi_d_SG_D_3_fdaf0), d_w_SG_D_3_block/3(State_psi_d_SG_D_3_b825f), T_e_SG_D_3_block/1(State_psi_d_SG_D_3_0515e), T_e_SG_D_3_block/7(State_psi_d_SG_D_3_355d2)
  d_psi_kq_SG_D_3_block/1(Blockout_d_psi_kq_SG_D_3_acb7b) -> psi_kq_SG_D_3/1
  psi_1d_SG_D_3/1 -> d_psi_fd_SG_D_3_block/3(State_psi_1d_SG_D_3_a842a), d_psi_fd_SG_D_3_block/5(State_psi_1d_SG_D_3_8aaf0), d_psi_fd_SG_D_3_block/8(State_psi_1d_SG_D_3_7f19e), d_psi_d_SG_D_3_block/1(State_psi_1d_SG_D_3_2013b), d_w_SG_D_3_block/8(State_psi_1d_SG_D_3_df021), d_V_f_SG_D_3_block/4(State_psi_1d_SG_D_3_fdc7a), i_d_SG_D_3_block/5(State_psi_1d_SG_D_3_ba81f), i_q_SG_D_3_block/5(State_psi_1d_SG_D_3_88e27), d_psi_1d_SG_D_3_block/1(State_psi_1d_SG_D_3_3b403), T_e_SG_D_3_block/6(State_psi_1d_SG_D_3_44396), d_psi_1d_SG_D_3_block/3(State_psi_1d_SG_D_3_4c72e)
  psi_q_SG_D_3/1 -> d_psi_d_SG_D_3_block/8(State_psi_q_SG_D_3_01c82), d_psi_gq_SG_D_3_block/6(State_psi_q_SG_D_3_d87f8), d_psi_gq_SG_D_3_block/9(State_psi_q_SG_D_3_0f8a4), d_psi_kq_SG_D_3_block/5(State_psi_q_SG_D_3_1522f), d_psi_q_SG_D_3_block/3(State_psi_q_SG_D_3_33284), d_V_f_SG_D_3_block/7(State_psi_q_SG_D_3_72b18), d_w_SG_D_3_block/6(State_psi_q_SG_D_3_c3d2e), d_V_f_SG_D_3_block/11(State_psi_q_SG_D_3_0b65f), i_d_SG_D_3_block/3(State_psi_q_SG_D_3_70eb0), i_q_SG_D_3_block/3(State_psi_q_SG_D_3_60de2), T_e_SG_D_3_block/4(State_psi_q_SG_D_3_52c06), d_w_SG_D_3_block/7(State_psi_q_SG_D_3_f932d), T_e_SG_D_3_block/5(State_psi_q_SG_D_3_d7233)
  psi_fd_SG_D_3/1 -> d_psi_fd_SG_D_3_block/2(State_psi_fd_SG_D_3_7ac4b), d_psi_fd_SG_D_3_block/4(State_psi_fd_SG_D_3_12a65), d_psi_fd_SG_D_3_block/10(State_psi_fd_SG_D_3_0d84b), d_psi_1d_SG_D_3_block/5(State_psi_fd_SG_D_3_649d9), d_psi_fd_SG_D_3_block/7(State_psi_fd_SG_D_3_2014a), d_w_SG_D_3_block/10(State_psi_fd_SG_D_3_b5ce7), d_V_f_SG_D_3_block/6(State_psi_fd_SG_D_3_cd25d), i_q_SG_D_3_block/7(State_psi_fd_SG_D_3_58217), d_psi_1d_SG_D_3_block/2(State_psi_fd_SG_D_3_f9b6a), d_psi_d_SG_D_3_block/3(State_psi_fd_SG_D_3_0e180), T_e_SG_D_3_block/8(State_psi_fd_SG_D_3_44178), i_d_SG_D_3_block/7(State_psi_fd_SG_D_3_ca9c0)
  psi_gq_SG_D_3/1 -> d_psi_q_SG_D_3_block/1(State_psi_gq_SG_D_3_1dddd), d_psi_gq_SG_D_3_block/1(State_psi_gq_SG_D_3_42abb), d_psi_gq_SG_D_3_block/2(State_psi_gq_SG_D_3_81b5d), d_psi_gq_SG_D_3_block/4(State_psi_gq_SG_D_3_55563), d_psi_kq_SG_D_3_block/3(State_psi_gq_SG_D_3_b2b08), d_w_SG_D_3_block/4(State_psi_gq_SG_D_3_617ad), d_V_f_SG_D_3_block/9(State_psi_gq_SG_D_3_47fb2), d_psi_gq_SG_D_3_block/7(State_psi_gq_SG_D_3_b3e08), i_d_SG_D_3_block/1(State_psi_gq_SG_D_3_83e92), i_q_SG_D_3_block/1(State_psi_gq_SG_D_3_e58b5), T_e_SG_D_3_block/2(State_psi_gq_SG_D_3_1cc94), d_psi_kq_SG_D_3_block/1(State_psi_gq_SG_D_3_4cb6a)
  theta_SG_D_3_out_block/1(Blockout_theta_SG_D_3_out_a9243) -> theta_SG_D_3_out/1
  d_V_f_SG_D_3_block/1(Blockout_d_V_f_SG_D_3_d48b4) -> V_f_SG_D_3/1
  i_d_SG_D_3_block/1(Blockout_i_d_SG_D_3_8b105) -> i_d_SG_D_3/1
  d_psi_d_SG_D_3_block/1(Blockout_d_psi_d_SG_D_3_27069) -> psi_d_SG_D_3/1
  i_q_SG_D_3_block/1(Blockout_i_q_SG_D_3_d37fb) -> i_q_SG_D_3/1
  d_psi_q_SG_D_3_block/1(Blockout_d_psi_q_SG_D_3_a4a1c) -> psi_q_SG_D_3/1
  d_R_f_SG_D_3_block/1(Blockout_d_R_f_SG_D_3_894a9) -> R_f_SG_D_3/1
  d_psi_1d_SG_D_3_block/1(Blockout_d_psi_1d_SG_D_3_0c79f) -> psi_1d_SG_D_3/1
  T_e_SG_D_3_block/1(Blockout_T_e_SG_D_3_5900b) -> T_e_SG_D_3/1
  d_psi_gq_SG_D_3_block/1(Blockout_d_psi_gq_SG_D_3_5066e) -> psi_gq_SG_D_3/1
  V_f_SG_D_3/1 -> d_V_f_SG_D_3_block/14(State_V_f_SG_D_3_66c81), d_E_fd_SG_D_3_block/2(State_V_f_SG_D_3_2af07)
  Px_3_SG_D_3/1 -> d_V_f_SG_D_3_block/3(State_Px_3_SG_D_3_a594e), d_Px_3_SG_D_3_block/1(State_Px_3_SG_D_3_2f57b)
  d_E_fd_SG_D_3_block/1(Blockout_d_E_fd_SG_D_3_8336f) -> E_fd_SG_D_3/1
  E_fd_SG_D_3/1 -> d_V_f_SG_D_3_block/1(State_E_fd_SG_D_3_5ffef), d_E_fd_SG_D_3_block/1(State_E_fd_SG_D_3_d3096), d_psi_fd_SG_D_3_block/1(State_E_fd_SG_D_3_c498c), d_R_f_SG_D_3_block/1(State_E_fd_SG_D_3_8b5d7)
  d_psi_fd_SG_D_3_block/1(Blockout_d_psi_fd_SG_D_3_9596e) -> psi_fd_SG_D_3/1

== system case5/AC_1/d_id_line_1_4_block ==
  note: d_id_line_1_4 in case5
      | $376.991118430775\,\mathrm{iq}_{\mathrm{line},1,4}+6332.81249201072\,\mathrm{vd}_{\mathrm{bus},1}-6332.81249201072\,\mathrm{vd}_{\mathrm{bus},4}$
      | Automatically generated on 2025-10-31 19:14:13 .
  State_iq_line_1_4_f9009 : Inport
  State_vd_bus_1_aee9d : Inport  Port=2
  State_vd_bus_4_1db4d : Inport  Port=3
  Add_ead1a : Sum
  Constant_376.991118430775_7df71 : Constant  Value=376.991118430775
  Constant_6332.81249201072_2a037 : Constant  Value=6332.81249201072
  Constant_6332.81249201072_2c4bb : Constant  Value=6332.81249201072
  Product_04931 : Product
  Product_4f94b : Product
  Product_907b6 : Product
  Subtract_c8ec4 : Sum  Inputs=+-
  Blockout_d_id_line_1_4_69e37 : Outport
  wires:
  Constant_376.991118430775_7df71/1 -> Product_907b6/1
  Product_4f94b/1 -> Add_ead1a/2
  State_iq_line_1_4_f9009/1 -> Product_907b6/2
  Subtract_c8ec4/1 -> Blockout_d_id_line_1_4_69e37/1
  Constant_6332.81249201072_2c4bb/1 -> Product_4f94b/1
  Product_907b6/1 -> Add_ead1a/1
  State_vd_bus_1_aee9d/1 -> Product_4f94b/2
  Constant_6332.81249201072_2a037/1 -> Product_04931/1
  State_vd_bus_4_1db4d/1 -> Product_04931/2
  Add_ead1a/1 -> Subtract_c8ec4/1
  Product_04931/1 -> Subtract_c8ec4/2

== system case5/AC_1/d_id_line_3_6_block ==
  note: d_id_line_3_6 in case5
      | $376.991118430775\,\mathrm{iq}_{\mathrm{line},3,6}+6224.74401945081\,\mathrm{vd}_{\mathrm{bus},3}-6224.74401945081\,\mathrm{vd}_{\mathrm{bus},6}$
      | Automatically generated on 2025-10-31 19:14:22 .
  State_iq_line_3_6_0028c : Inport
  State_vd_bus_3_b4f76 : Inport  Port=2
  State_vd_bus_6_aaa66 : Inport  Port=3
  Add_fe0f0 : Sum
  Constant_376.991118430775_66f8f : Constant  Value=376.991118430775
  Constant_6224.74401945081_f6c00 : Constant  Value=6224.74401945081
  Constant_6224.74401945081_fa8d3 : Constant  Value=6224.74401945081
  Product_20f8b : Product
  Product_2217c : Product
  Product_6d514 : Product
  Subtract_a8b68 : Sum  Inputs=+-
  Blockout_d_id_line_3_6_09483 : Outport
  wires:
  State_vd_bus_3_b4f76/1 -> Product_2217c/2
  Constant_376.991118430775_66f8f/1 -> Product_6d514/1
  Product_2217c/1 -> Add_fe0f0/2
  State_iq_line_3_6_0028c/1 -> Product_6d514/2
  Constant_6224.74401945081_f6c00/1 -> Product_2217c/1
  Product_6d514/1 -> Add_fe0f0/1
  Constant_6224.74401945081_fa8d3/1 -> Product_20f8b/1
  State_vd_bus_6_aaa66/1 -> Product_20f8b/2
  Add_fe0f0/1 -> Subtract_a8b68/1
  Product_20f8b/1 -> Subtract_a8b68/2
  Subtract_a8b68/1 -> Blockout_d_id_line_3_6_09483/1

== system case5/AC_1/d_id_line_4_5_block ==
  note: d_id_line_4_5 in case5
      | $376.991118430775\,\mathrm{iq}_{\mathrm{line},4,5}-65.6746171008477\,\mathrm{id}_{\mathrm{line},4,5}+3964.89129934584\,\mathrm{vd}_{\mathrm{bus},4}-3964.89129934584\,\mathrm{vd}_{\mathrm{bus},5}$
      | Automatically generated on 2025-10-31 19:14:16 .
  State_id_line_4_5_17bd4 : Inport
  State_iq_line_4_5_655b9 : Inport  Port=2
  State_vd_bus_4_6c299 : Inport  Port=3
  State_vd_bus_5_8ddf9 : Inport  Port=4
  Add_c2b6e : Sum
  Add_d47a9 : Sum
  Constant_-65.6746171008477_39d8a : Constant  Value=-65.6746171008477
  Constant_376.991118430775_7b4b7 : Constant  Value=376.991118430775
  Constant_3964.89129934584_47147 : Constant  Value=3964.89129934584
  Constant_3964.89129934584_8503d : Constant  Value=3964.89129934584
  Product_2368b : Product
  Product_ac17c : Product
  Product_af8bf : Product
  Product_cb9f4 : Product
  Subtract_c96c4 : Sum  Inputs=+-
  Blockout_d_id_line_4_5_8120d : Outport
  wires:
  Constant_-65.6746171008477_39d8a/1 -> Product_2368b/1
  Product_af8bf/1 -> Add_d47a9/2
  State_id_line_4_5_17bd4/1 -> Product_2368b/2
  Constant_376.991118430775_7b4b7/1 -> Product_af8bf/1
  State_iq_line_4_5_655b9/1 -> Product_af8bf/2
  Product_2368b/1 -> Add_d47a9/1
  Constant_3964.89129934584_47147/1 -> Product_cb9f4/1
  State_vd_bus_4_6c299/1 -> Product_cb9f4/2
  Add_d47a9/1 -> Add_c2b6e/1
  Product_cb9f4/1 -> Add_c2b6e/2
  Constant_3964.89129934584_8503d/1 -> Product_ac17c/1
  State_vd_bus_5_8ddf9/1 -> Product_ac17c/2
  Add_c2b6e/1 -> Subtract_c96c4/1
  Product_ac17c/1 -> Subtract_c96c4/2
  Subtract_c96c4/1 -> Blockout_d_id_line_4_5_8120d/1

== system case5/AC_1/d_id_line_5_6_block ==
  note: d_id_line_5_6 in case5
      | $376.991118430775\,\mathrm{iq}_{\mathrm{line},5,6}-81.5365142414676\,\mathrm{id}_{\mathrm{line},5,6}+2145.70587964598\,\mathrm{vd}_{\mathrm{bus},5}-2145.70587964598\,\mathrm{vd}_{\mathrm{bus},6}$
      | Automatically generated on 2025-10-31 19:14:20 .
  State_id_line_5_6_f0fe5 : Inport
  State_iq_line_5_6_2c004 : Inport  Port=2
  State_vd_bus_5_7c77b : Inport  Port=3
  State_vd_bus_6_16423 : Inport  Port=4
  Add_9cd58 : Sum
  Add_d995d : Sum
  Constant_-81.5365142414676_467ac : Constant  Value=-81.5365142414676
  Constant_2145.70587964598_1dc87 : Constant  Value=2145.70587964598
  Constant_2145.70587964598_55cfb : Constant  Value=2145.70587964598
  Constant_376.991118430775_9207b : Constant  Value=376.991118430775
  Product_5cdd8 : Product
  Product_965fc : Product
  Product_c4f28 : Product
  Product_cd52a : Product
  Subtract_9e544 : Sum  Inputs=+-
  Blockout_d_id_line_5_6_90114 : Outport
  wires:
  Constant_-81.5365142414676_467ac/1 -> Product_cd52a/1
  Product_c4f28/1 -> Add_d995d/2
  State_id_line_5_6_f0fe5/1 -> Product_cd52a/2
  Constant_376.991118430775_9207b/1 -> Product_c4f28/1
  Product_cd52a/1 -> Add_d995d/1
  State_iq_line_5_6_2c004/1 -> Product_c4f28/2
  Constant_2145.70587964598_55cfb/1 -> Product_965fc/1
  Product_5cdd8/1 -> Subtract_9e544/2
  State_vd_bus_5_7c77b/1 -> Product_965fc/2
  Add_d995d/1 -> Add_9cd58/1
  Product_965fc/1 -> Add_9cd58/2
  Constant_2145.70587964598_1dc87/1 -> Product_5cdd8/1
  State_vd_bus_6_16423/1 -> Product_5cdd8/2
  Add_9cd58/1 -> Subtract_9e544/1
  Subtract_9e544/1 -> Blockout_d_id_line_5_6_90114/1

== system case5/AC_1/d_id_line_6_7_block ==
  note: d_id_line_6_7 in case5
      | $376.991118430775\,\mathrm{iq}_{\mathrm{line},6,7}-41.9587831477638\,\mathrm{id}_{\mathrm{line},6,7}+3618.7499954347\,\mathrm{vd}_{\mathrm{bus},6}-3618.7499954347\,\mathrm{vd}_{\mathrm{bus},7}$
      | Automatically generated on 2025-10-31 19:14:26 .
  State_id_line_6_7_b019b : Inport
  State_iq_line_6_7_c30b7 : Inport  Port=2
  State_vd_bus_6_ae47b : Inport  Port=3
  State_vd_bus_7_eaeb2 : Inport  Port=4
  Add_3454d : Sum
  Add_e198f : Sum
  Constant_-41.9587831477638_a3320 : Constant  Value=-41.9587831477638
  Constant_3618.7499954347_27d84 : Constant  Value=3618.7499954347
  Constant_3618.7499954347_ffe82 : Constant  Value=3618.7499954347
  Constant_376.991118430775_67dcd : Constant  Value=376.991118430775
  Product_1b772 : Product
  Product_1f7c2 : Product
  Product_9817c : Product
  Product_f6d09 : Product
  Subtract_b73b8 : Sum  Inputs=+-
  Blockout_d_id_line_6_7_ed3ed : Outport
  wires:
  Constant_-41.9587831477638_a3320/1 -> Product_1f7c2/1
  Product_f6d09/1 -> Add_e198f/2
  State_id_line_6_7_b019b/1 -> Product_1f7c2/2
  Constant_376.991118430775_67dcd/1 -> Product_f6d09/1
  State_iq_line_6_7_c30b7/1 -> Product_f6d09/2
  Product_1f7c2/1 -> Add_e198f/1
  Constant_3618.7499954347_ffe82/1 -> Product_9817c/1
  State_vd_bus_6_ae47b/1 -> Product_9817c/2
  Add_e198f/1 -> Add_3454d/1
  Product_9817c/1 -> Add_3454d/2
  Constant_3618.7499954347_27d84/1 -> Product_1b772/1
  State_vd_bus_7_eaeb2/1 -> Product_1b772/2
  Add_3454d/1 -> Subtract_b73b8/1
  Product_1b772/1 -> Subtract_b73b8/2
  Subtract_b73b8/1 -> Blockout_d_id_line_6_7_ed3ed/1

== system case5/AC_1/d_id_line_7_8_block ==
  note: d_id_line_7_8 in case5
      | $376.991118430775\,\mathrm{iq}_{\mathrm{line},7,8}-41.9587831477638\,\mathrm{id}_{\mathrm{line},7,8}+5066.24999360857\,\mathrm{vd}_{\mathrm{bus},7}-5066.24999360857\,\mathrm{vd}_{\mathrm{bus},8}$
      | Automatically generated on 2025-10-31 19:14:29 .
  State_id_line_7_8_e67d2 : Inport
  State_iq_line_7_8_154d0 : Inport  Port=2
  State_vd_bus_7_5624b : Inport  Port=3
  State_vd_bus_8_a9172 : Inport  Port=4
  Add_728fb : Sum
  Add_e1eba : Sum
  Constant_-41.9587831477638_a6fab : Constant  Value=-41.9587831477638
  Constant_376.991118430775_68c3a : Constant  Value=376.991118430775
  Constant_5066.24999360857_6dca0 : Constant  Value=5066.24999360857
  Constant_5066.24999360857_943c5 : Constant  Value=5066.24999360857
  Product_04255 : Product
  Product_494e5 : Product
  Product_a82e5 : Product
  Product_f289f : Product
  Subtract_8760c : Sum  Inputs=+-
  Blockout_d_id_line_7_8_f2a9f : Outport
  wires:
  Constant_-41.9587831477638_a6fab/1 -> Product_a82e5/1
  Product_04255/1 -> Add_728fb/2
  State_id_line_7_8_e67d2/1 -> Product_a82e5/2
  Constant_376.991118430775_68c3a/1 -> Product_04255/1
  Product_a82e5/1 -> Add_728fb/1
  State_iq_line_7_8_154d0/1 -> Product_04255/2
  Constant_5066.24999360857_943c5/1 -> Product_f289f/1
  State_vd_bus_7_5624b/1 -> Product_f289f/2
  Add_728fb/1 -> Add_e1eba/1
  Product_f289f/1 -> Add_e1eba/2
  Constant_5066.24999360857_6dca0/1 -> Product_494e5/1
  State_vd_bus_8_a9172/1 -> Product_494e5/2
  Add_e1eba/1 -> Subtract_8760c/1
  Product_494e5/1 -> Subtract_8760c/2
  Subtract_8760c/1 -> Blockout_d_id_line_7_8_f2a9f/1

== system case5/AC_1/d_id_line_8_2_block ==
  note: d_id_line_8_2 in case5
      | $376.991118430775\,\mathrm{iq}_{\mathrm{line},8,2}-5836.31999263708\,\mathrm{vd}_{\mathrm{bus},2}+5836.31999263708\,\mathrm{vd}_{\mathrm{bus},8}$
      | Automatically generated on 2025-10-31 19:14:33 .
  State_iq_line_8_2_968c6 : Inport
  State_vd_bus_2_be716 : Inport  Port=2
  State_vd_bus_8_d36f6 : Inport  Port=3
  Add_a13d2 : Sum
  Constant_376.991118430775_15e6d : Constant  Value=376.991118430775
  Constant_5836.31999263708_09253 : Constant  Value=5836.31999263708
  Constant_5836.31999263708_d98ef : Constant  Value=5836.31999263708
  Product_35f16 : Product
  Product_6c7a6 : Product
  Product_d570d : Product
  Subtract_683f5 : Sum  Inputs=+-
  Blockout_d_id_line_8_2_55ace : Outport
  wires:
  State_vd_bus_2_be716/1 -> Product_6c7a6/2
  Constant_376.991118430775_15e6d/1 -> Product_d570d/1
  Product_6c7a6/1 -> Subtract_683f5/2
  State_iq_line_8_2_968c6/1 -> Product_d570d/2
  Constant_5836.31999263708_09253/1 -> Product_6c7a6/1
  Product_d570d/1 -> Subtract_683f5/1
  Constant_5836.31999263708_d98ef/1 -> Product_35f16/1
  State_vd_bus_8_d36f6/1 -> Product_35f16/2
  Subtract_683f5/1 -> Add_a13d2/1
  Product_35f16/1 -> Add_a13d2/2
  Add_a13d2/1 -> Blockout_d_id_line_8_2_55ace/1

== system case5/AC_1/d_id_line_8_9_block ==
  note: d_id_line_8_9 in case5
      | $376.991118430775\,\mathrm{iq}_{\mathrm{line},8,9}-70.6416049488109\,\mathrm{id}_{\mathrm{line},8,9}+2265.65217105477\,\mathrm{vd}_{\mathrm{bus},8}-2265.65217105477\,\mathrm{vd}_{\mathrm{bus},9}$
      | Automatically generated on 2025-10-31 19:14:36 .
  State_id_line_8_9_f8c14 : Inport
  State_iq_line_8_9_03554 : Inport  Port=2
  State_vd_bus_8_1c687 : Inport  Port=3
  State_vd_bus_9_9fd7e : Inport  Port=4
  Add_a4439 : Sum
  Add_ce1b3 : Sum
  Constant_-70.6416049488109_91976 : Constant  Value=-70.6416049488109
  Constant_2265.65217105477_7654a : Constant  Value=2265.65217105477
  Constant_2265.65217105477_c045e : Constant  Value=2265.65217105477
  Constant_376.991118430775_a6ec5 : Constant  Value=376.991118430775
  Product_9e57b : Product
  Product_b0d93 : Product
  Product_fc98a : Product
  Product_fe1e7 : Product
  Subtract_81de5 : Sum  Inputs=+-
  Blockout_d_id_line_8_9_41799 : Outport
  wires:
  Constant_-70.6416049488109_91976/1 -> Product_9e57b/1
  Product_fc98a/1 -> Add_ce1b3/2
  State_id_line_8_9_f8c14/1 -> Product_9e57b/2
  Constant_376.991118430775_a6ec5/1 -> Product_fc98a/1
  State_iq_line_8_9_03554/1 -> Product_fc98a/2
  Product_9e57b/1 -> Add_ce1b3/1
  Constant_2265.65217105477_c045e/1 -> Product_b0d93/1
  State_vd_bus_8_1c687/1 -> Product_b0d93/2
  Add_ce1b3/1 -> Add_a4439/1
  Product_b0d93/1 -> Add_a4439/2
  Constant_2265.65217105477_7654a/1 -> Product_fe1e7/1
  State_vd_bus_9_9fd7e/1 -> Product_fe1e7/2
  Add_a4439/1 -> Subtract_81de5/1
  Product_fe1e7/1 -> Subtract_81de5/2
  Subtract_81de5/1 -> Blockout_d_id_line_8_9_41799/1

== system case5/AC_1/d_id_line_9_4_block ==
  note: d_id_line_9_4 in case5
      | $376.991118430775\,\mathrm{iq}_{\mathrm{line},9,4}-41.8135970469065\,\mathrm{id}_{\mathrm{line},9,4}-4291.41175929197\,\mathrm{vd}_{\mathrm{bus},4}+4291.41175929197\,\mathrm{vd}_{\mathrm{bus},9}$
      | Automatically generated on 2025-10-31 19:14:40 .
  State_id_line_9_4_837f3 : Inport
  State_iq_line_9_4_dc97c : Inport  Port=2
  State_vd_bus_4_e4399 : Inport  Port=3
  State_vd_bus_9_b8585 : Inport  Port=4
  Add_47ed7 : Sum
  Add_7d07b : Sum
  Constant_-41.8135970469065_ae39a : Constant  Value=-41.8135970469065
  Constant_376.991118430775_5896f : Constant  Value=376.991118430775
  Constant_4291.41175929197_18d57 : Constant  Value=4291.41175929197
  Constant_4291.41175929197_e7ca9 : Constant  Value=4291.41175929197
  Product_3c9c7 : Product
  Product_41d74 : Product
  Product_63c9a : Product
  Product_d23df : Product
  Subtract_a9f16 : Sum  Inputs=+-
  Blockout_d_id_line_9_4_0af09 : Outport
  wires:
  Constant_-41.8135970469065_ae39a/1 -> Product_41d74/1
  Product_63c9a/1 -> Add_7d07b/2
  State_id_line_9_4_837f3/1 -> Product_41d74/2
  Constant_376.991118430775_5896f/1 -> Product_63c9a/1
  Product_41d74/1 -> Add_7d07b/1
  State_iq_line_9_4_dc97c/1 -> Product_63c9a/2
  Constant_4291.41175929197_e7ca9/1 -> Product_3c9c7/1
  State_vd_bus_4_e4399/1 -> Product_3c9c7/2
  Add_7d07b/1 -> Subtract_a9f16/1
  Product_3c9c7/1 -> Subtract_a9f16/2
  Constant_4291.41175929197_18d57/1 -> Product_d23df/1
  Subtract_a9f16/1 -> Add_47ed7/1
  State_vd_bus_9_b8585/1 -> Product_d23df/2
  Product_d23df/1 -> Add_47ed7/2
  Add_47ed7/1 -> Blockout_d_id_line_9_4_0af09/1

== system case5/AC_1/d_id_load_5_block ==
  note: d_id_load_5 in case5
      | $376.991118430775\,\mathrm{iq}_{\mathrm{load},5}-1083.07680322081\,\mathrm{id}_{\mathrm{load},5}+1127.5659037617\,\mathrm{vd}_{\mathrm{bus},5}$
      | Automatically generated on 2025-10-31 19:14:04 .
  State_id_load_5_4be11 : Inport
  State_iq_load_5_a5206 : Inport  Port=2
  State_vd_bus_5_53255 : Inport  Port=3
  Add_18e09 : Sum
  Add_b9a49 : Sum
  Constant_-1083.07680322081_1dfb8 : Constant  Value=-1083.07680322081
  Constant_1127.5659037617_b6c0d : Constant  Value=1127.5659037617
  Constant_376.991118430775_8d0a8 : Constant  Value=376.991118430775
  Product_23679 : Product
  Product_34619 : Product
  Product_51c62 : Product
  Blockout_d_id_load_5_989b8 : Outport
  wires:
  Constant_-1083.07680322081_1dfb8/1 -> Product_51c62/1
  Product_23679/1 -> Add_18e09/2
  State_id_load_5_4be11/1 -> Product_51c62/2
  Constant_376.991118430775_8d0a8/1 -> Product_23679/1
  Product_34619/1 -> Add_b9a49/2
  State_iq_load_5_a5206/1 -> Product_23679/2
  Product_51c62/1 -> Add_18e09/1
  Constant_1127.5659037617_b6c0d/1 -> Product_34619/1
  State_vd_bus_5_53255/1 -> Product_34619/2
  Add_18e09/1 -> Add_b9a49/1
  Add_b9a49/1 -> Blockout_d_id_load_5_989b8/1
